simulink model "Plataforma"  (R2015b)
settings: Solver=ode45  StartTime=0.0  StopTime=tf  MaxStep=1e-1  RelTol=1e-3  AbsTol=1e-3
InitFcn:
  | c = clock;
  | seed_offset = c(6);
  | seed_offset = floor(seed_offset);
undefined symbols (not defined in the file): Ts
libraries: vrlib x4
settings Model: Creator=Davi  LastModifiedBy=juliocvidal
settings DataIOCC: SaveFormat=Array  SignalLoggingSaveFormat=ModelDataLogs
settings OptimizationCC: ExpressionDepthLimit=2147483647
settings DebuggingCC: UnderspecifiedInitializationDetection=Classic  MergeDetectMultiDrivingBlocksExec=none  SolverPrmCheckMsg=warning  InheritedTsInSrcMsg=none  FcnCallInpInsideContextMsg=EnableAllAsWarning  AllowSymbolicDim=on  StateNameClashWarn=warning
settings HardwareCC: ProdBitPerPointer=32  ProdLargestAtomicFloat=None  ProdIntDivRoundTo=Undefined  ProdEndianess=Unspecified  ProdWordSize=32  ProdHWDeviceType=32-bit Generic
settings GRTTargetCC: GeneratePreprocessorConditionals=Disable all
settings ConfigComp: CovModelRefEnable=Off

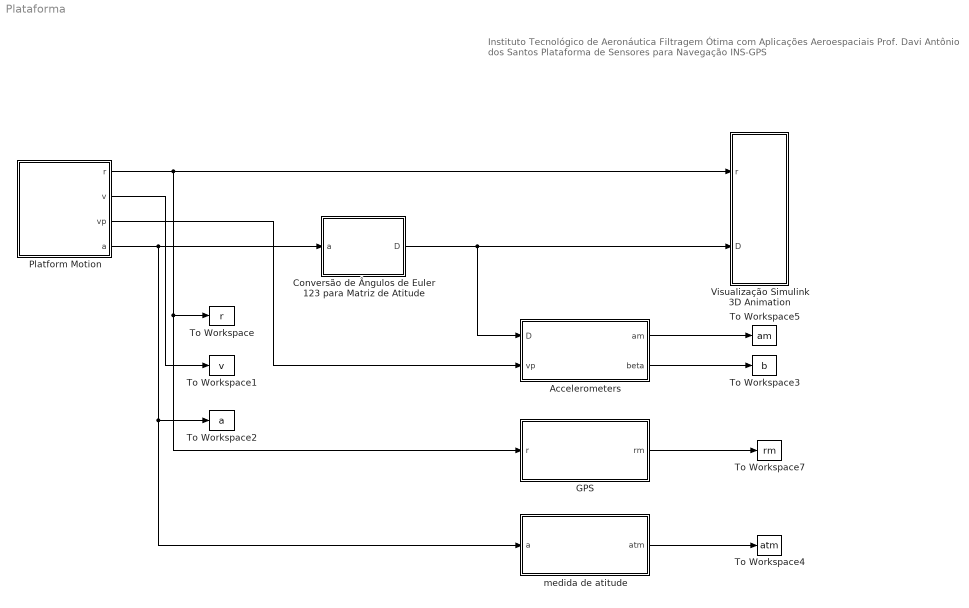
== system Plataforma ==
  note: Instituto Tecnológico de Aeronáutica
      | Filtragem Ótima com Aplicações Aeroespaciais
      | Prof. Davi Antônio dos Santos
      |
      | Plataforma de Sensores para Navegação INS-GPS
  Accelerometers : Subsystem  mask{beta=[0.1 -0.1 0.2]', sigma_i=0.0039, sigma_b=0.001, seed=1+seed_offset}
      mask prompts: beta "Bias (beta)"; sigma_i "Desvio padrão do ruído (sigma_i)"; sigma_b "Desvio padrão bias (sigma_b)"
  Conversão de Ângulos de Euler 123 para Matriz de Atitude : MATLAB Function  TreatAsAtomicUnit=on
  GPS : Subsystem  mask{sigma=1, seed=2+seed_offset}
      mask prompts: sigma "Dev. padrão do ruído (sigma)"
  Platform Motion : Subsystem
  To Workspace : ToWorkspace  VariableName=r  SaveFormat=Structure With Time  SampleTime=Ts
  To Workspace1 : ToWorkspace  VariableName=v  SaveFormat=Structure With Time  SampleTime=Ts
  To Workspace2 : ToWorkspace  VariableName=a  SaveFormat=Structure With Time  SampleTime=Ts
  To Workspace3 : ToWorkspace  VariableName=b  SaveFormat=Structure With Time  SampleTime=Ts
  To Workspace4 : ToWorkspace  VariableName=atm  SaveFormat=Structure With Time  SampleTime=Ts
  To Workspace5 : ToWorkspace  VariableName=am  SaveFormat=Structure With Time  SampleTime=Ts
  To Workspace7 : ToWorkspace  VariableName=rm  SaveFormat=Structure With Time  SampleTime=Ts
  Visualização Simulink 3D Animation : Subsystem
  medida de atitude : Subsystem  mask{sigma=0.035*0.1, seed=3+seed_offset}
      mask prompts: sigma "Dev. padrão do ruído (sigma)"
  wires:
  Platform Motion/4(a) -> Conversão de Ângulos de Euler 123 para Matriz de Atitude/1(a), medida de atitude/1(a), To Workspace2/1
  Platform Motion/3(vp) -> Accelerometers/2(vp)
  Platform Motion/2(v) -> To Workspace1/1
  Accelerometers/2(beta) -> To Workspace3/1
  Accelerometers/1(am) -> To Workspace5/1
  GPS/1(rm) -> To Workspace7/1
  Platform Motion/1(r) -> GPS/1(r), To Workspace/1, Visualização Simulink 3D Animation/1(r)
  Conversão de Ângulos de Euler 123 para Matriz de Atitude/1(D) -> Accelerometers/1(D), Visualização Simulink 3D Animation/2(D)
  medida de atitude/1(atm) -> To Workspace4/1

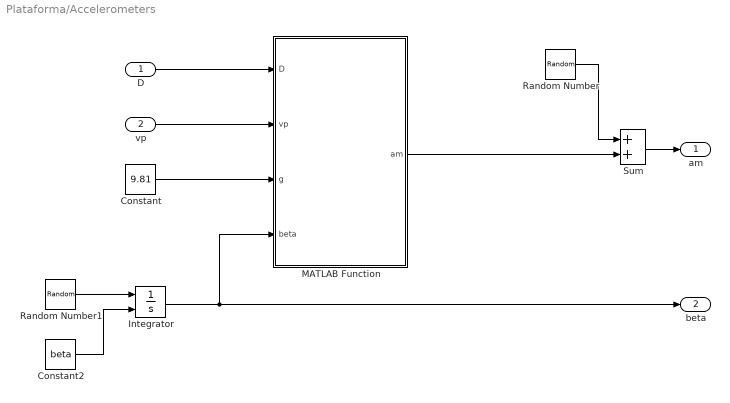
== system Plataforma/Accelerometers ==
  D : Inport
  vp : Inport  Port=2
  Constant : Constant  Value=9.81
  Constant2 : Constant  Value=beta
  Integrator : Integrator  InitialConditionSource=external
  MATLAB Function : MATLAB Function  TreatAsAtomicUnit=on
  Random Number : RandomNumber  Mean=[0 0 0]'  Variance="[sigma_i^2  sigma_i^2  sigma_i^2]'"  Seed=seed
  Random Number1 : RandomNumber  Mean=[0 0 0]'  Variance="[sigma_b^2  sigma_b^2  sigma_b^2]'"  Seed=seed+1
  Sum : Sum
  am : Outport
  beta : Outport  Port=2
  wires:
  D/1 -> MATLAB Function/1(D)
  vp/1 -> MATLAB Function/2(vp)
  MATLAB Function/1(am) -> Sum/2
  Constant/1 -> MATLAB Function/3(g)
  Random Number/1 -> Sum/1
  Sum/1 -> am/1
  Constant2/1 -> Integrator/2
  Integrator/1 -> MATLAB Function/4(beta), beta/1
  Random Number1/1 -> Integrator/1

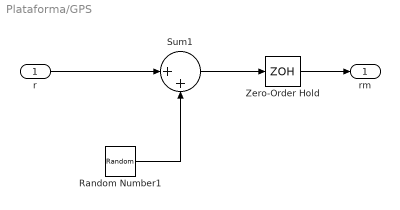
== system Plataforma/GPS ==
  r : Inport
  Random Number1 : RandomNumber  Mean=[0 0 0]'  Variance="[sigma^2  sigma^2  sigma^2]'"  Seed=seed
  Sum1 : Sum  Inputs=|++
  Zero-Order Hold : ZeroOrderHold  SampleTime=0.1
  rm : Outport
  wires:
  r/1 -> Sum1/1
  Random Number1/1 -> Sum1/2
  Sum1/1 -> Zero-Order Hold/1
  Zero-Order Hold/1 -> rm/1

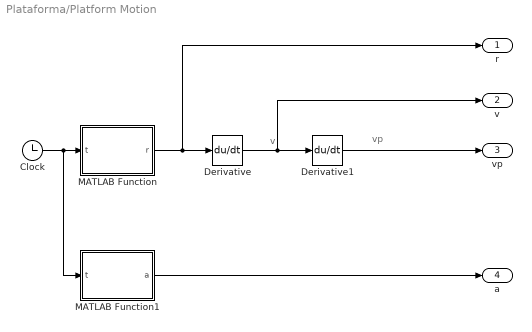
== system Plataforma/Platform Motion ==
  note: vp
  note: v
  Clock : Clock
  Derivative : Derivative
  Derivative1 : Derivative
  MATLAB Function : MATLAB Function  TreatAsAtomicUnit=on
  MATLAB Function1 : MATLAB Function  TreatAsAtomicUnit=on
  r : Outport
  v : Outport  Port=2
  vp : Outport  Port=3
  a : Outport  Port=4
  wires:
  Clock/1 -> MATLAB Function1/1(t), MATLAB Function/1(t)
  Derivative1/1 -> vp/1
  MATLAB Function1/1(a) -> a/1
  Derivative/1 -> v/1, Derivative1/1
  MATLAB Function/1(r) -> r/1, Derivative/1

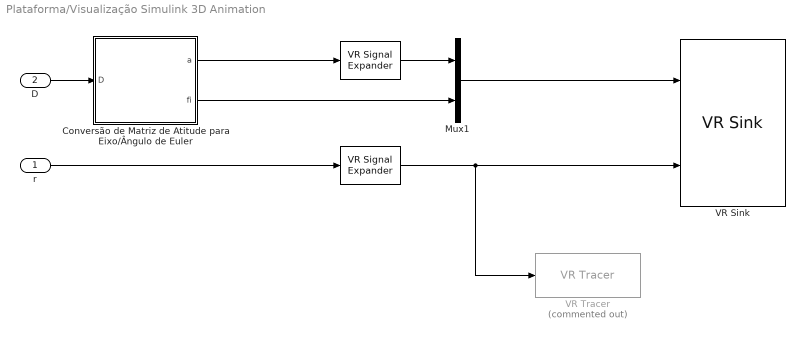
== system Plataforma/Visualização Simulink 3D Animation ==
  r : Inport
  D : Inport  Port=2
  "    " : vrlib/VR Signal Expander  outwidth=3  outidx=[3 1 2]
  "      " : vrlib/VR Signal Expander  outwidth=3  outidx=[3 1 2]
  Conversão de Matriz de Atitude para Eixo/Ângulo de Euler : MATLAB Function  TreatAsAtomicUnit=on
  Mux1 : Mux  Inputs=2
  VR Sink : vrlib/VR Sink  InstantiateOnLoad=on  SampleTime=-1  ViewEnable=on  RemoteChange=off  RemoteView=off  FieldsWritten=Quadrotor.rotation.4.1.1.double#Quadrotor.translation.3.1.1.double  WorldFileName=Quadricopter.WRL  AutoView=on  VideoDimensions=[]  AllowVariableSize=off  FigureProperties="{'Position', 'Name', 'Viewpoint', 'CameraBound', 'CameraDirection', 'CameraPosition', 'CameraUpVector', 'ZoomFactor', 'Antialiasing', 'Headlight', 'Lighting', 'NavPanel', 'Sound', 'StatusBar', 'Stereo3D', 'Stereo3DCameraOffset', 'Stereo3DHIT', 'ToolBar', 'Textures', 'Transparency', 'Triad', 'Wireframe', 'NavZones', 'NavMode', 'NavSpeed', 'CaptureFileFormat', 'CaptureFileName', 'Record2DCompressMethod', 'Record2DCompressQuality', 'Record2D', 'Record2DFileName', 'Record2DFPS'; [5.0000000000000000e+00   9.2333333333333371e+01   5.7600000000000000e+02   3.5000000000000000e+02], '', 'Top', 'on', [0.0000000000000000e+00   0.0000000000000000e+00  -1.0000000000000000e+00], [0.0000000000000000e+00   0.0000000000000000e+00   0.0000000000000000e+00], [0.0000000000000000e+00   1.0000000000000000e+00   0.0000000000000000e+00], [1.0000000000000000e+00], 'on', 'on', 'on', 'halfbar', 'on', 'on', 'off', [1.0000000149011612e-01], [0.0000000000000000e+00], 'on', 'on', 'on', 'none', 'off', 'off', 'fly', 'normal', 'tif', '%f_anim_%n.tif', 'auto', [7.5000000000000000e+01], 'off', '%f_anim_%n.avi', 'auto'}"
  VR Tracer : vrlib/VR Tracer  Commented=on  VrmlFile=Quadricopter.WRL  MarkerName=Tetrahedron  UseLines=on  UseTriads=on  MarkerScale=[0.03 0.03 0.03]  MarkerColorSelection=Selected from color list  MarkerColor=red  rgbval=[1 0 0]  Ts=0.5  ForceViewerOpen=off  ConnectPlane=off  PlaneCoeff=[0 1 0 0]  ConnectPoint=None  PointCoord=[0 0 0]
  wires:
  "      "/1 -> VR Sink/2, VR Tracer/1
  Mux1/1 -> VR Sink/1
  "    "/1 -> Mux1/1
  Conversão de Matriz de Atitude para Eixo/Ângulo de Euler/1(a) -> "    "/1
  Conversão de Matriz de Atitude para Eixo/Ângulo de Euler/2(fi) -> Mux1/2
  D/1 -> Conversão de Matriz de Atitude para Eixo/Ângulo de Euler/1(D)
  r/1 -> "      "/1

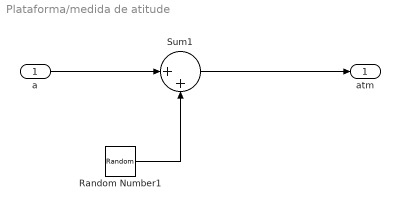
== system Plataforma/medida de atitude ==
  a : Inport
  Random Number1 : RandomNumber  Mean=[0 0 0]'  Variance="[sigma^2  sigma^2  sigma^2]'"  Seed=seed
  Sum1 : Sum  Inputs=|++
  atm : Outport
  wires:
  a/1 -> Sum1/1
  Random Number1/1 -> Sum1/2
  Sum1/1 -> atm/1

== matlab function Plataforma/Platform Motion/MATLAB Function ==
  data: t input; r output
function r = position(t)
%#codegen

% trajectória de posição, em S_R, em metros

Ax = 10;
Ay = 10;
Az = 1;
h = 20;


r = [Ax*sin(2*pi/20*t);
     Ay*cos(2*pi/20*t);
     Az*sin(2*pi/4*t) + h];

== matlab function Plataforma/Platform Motion/MATLAB Function1 ==
  data: t input; a output
function a = attitude(t)
%#codegen

% trajectória de atitude de S_P em relação a S_R, em rad

Afi = pi/18;
Ateta = pi/18;
Apsi = pi/18;

a = [Afi*sin(2*pi/2*t);
     Ateta*cos(2*pi/2*t);
     Apsi*sin(2*pi/8*t)];

== matlab function Plataforma/Visualização Simulink 3D Animation/Conversão de Matriz de Atitude para Eixo//Ângulo de Euler ==
  data: a output; D input; fi output
function [a,fi]  = D2afi(D)

% conversão de eixo/ângulo de Euler (fi,a) para matriz de atitude D

tr = trace(D);
cosseno = 0.5*(tr-1);
if abs(cosseno)>1, cosseno = sign(cosseno); end
fi = acos(cosseno);
a = zeros(3,1);

if tr==3,
    'a indefinido';
    a = [1 0 0]';
end

if tr==-1,
    
    s12 = sign(D(1,2));
    s23 = sign(D(2,3));
    
    s1 = 1;
    s2 = s12;
    s3 = s23*s2;
    
    a(1)= s1*sqrt(0.5*(1+D(1,1)));
    a(2)= s2*sqrt(0.5*(1+D(2,2)));
    a(3)= s3*sqrt(0.5*(1+D(3,3)));
end


if tr~=3 && tr~=-1,
   a(1) = (D(2,3)-D(3,2))/(2*sin(fi));
   a(2) = (D(3,1)-D(1,3))/(2*sin(fi));
   a(3) = (D(1,2)-D(2,1))/(2*sin(fi));
end

== matlab function Plataforma/Accelerometers/MATLAB Function ==
  data: D input; am output; vp input; g input; beta input
function am = fcn(D,vp,g,beta)
%#codegen

g_R = [0;0;-g];

am = D*(vp - g_R) + beta;

== matlab function Plataforma/Conversão de Ângulos de Euler 123 para Matriz de Atitude ==
  data: a input; D output
function D  = a1232D(a)

phi = a(1);
theta = a(2);
psi = a(3);

% conversão de ângulos de Euler 123 para matriz de atitude D

D = [cos(psi)*cos(theta), cos(psi)*sin(theta)*sin(phi)+sin(psi)*cos(phi), -cos(psi)*sin(theta)*cos(phi)+sin(psi)*sin(phi);
    -sin(psi)*cos(theta), -sin(psi)*sin(theta)*sin(phi)+cos(psi)*cos(phi), sin(psi)*sin(theta)*cos(phi)+cos(psi)*sin(phi);
    sin(theta) , -cos(theta)*sin(phi), cos(theta)*cos(phi)];
